simulink model "TPGCI_control_Simulation"  (R2024a)
settings: Solver=ode4  StartTime=0.0  StopTime=5  FixedStep=1e-6  RelTol=1e-3
undefined symbols (not defined in the file): DiscIntNeverNeededParam
libraries: slpidlib x3, spsThreePhaseSeriesRLCBranchLib x2, spsThreePhaseVIMeasurementLib x2, spsabctodq0Lib x2, spsDCVoltageSourceLib x1, spsGroundLib x1, spsPWMGenerator2LevelLib x1, spsThreePhaseParallelRLCBranchLib x1, spsThreePhaseSourceLib x1, spsUniversalBridgeLib x1, spsVoltageMeasurementLib x1, spsdq0toabcLib x1
settings Model: Creator=mahes  LastModifiedBy=mahes

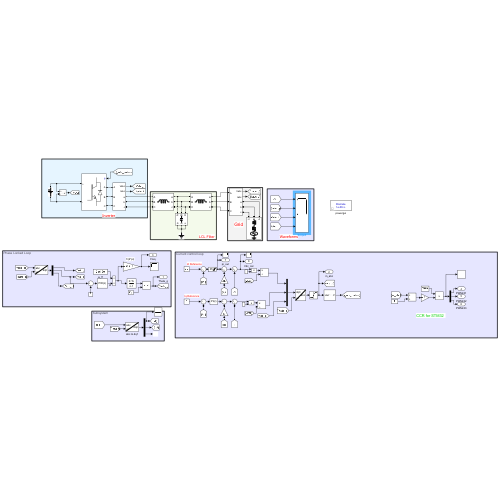
[thumbnail: Simulink's stored preview of the top-level diagram]
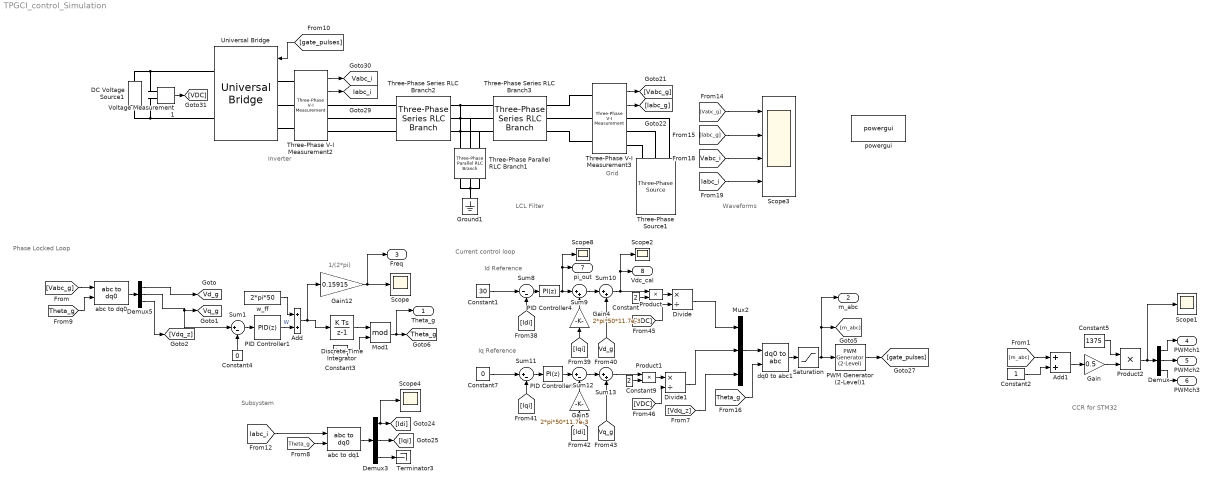
== system TPGCI_control_Simulation ==
  note: Subsystem
  note: Current control loop
  note: 1/(2*pi)
  note: Phase Locked Loop
  note: Grid
  note: Inverter
  note: Waveforms
  note: LCL Filter
  note: Id Reference
  note: Iq Reference
  note: CCR for STM32
  Add : Sum
  Add1 : Sum
  Constant : Constant  Value=2
  Constant1 : Constant  Value=30
  Constant2 : Constant
  Constant3 : Constant  Value=2*pi
  Constant4 : Constant  Value=0
  Constant5 : Constant  Value=1375
  Constant7 : Constant  Value=0
  Constant9 : Constant  Value=2
  DC Voltage Source1 : spsDCVoltageSourceLib/DC Voltage Source  Amplitude=800  Measurements=None
  Demux : Demux  Outputs=3
  Demux3 : Demux  Outputs=3
  Demux5 : Demux  Outputs=3
  Discrete-Time Integrator : DiscreteIntegrator  SampleTime=2e-5  ICPrevOutput=DiscIntNeverNeededParam  ICPrevScaledInput=DiscIntNeverNeededParam
  Divide : Product  Inputs=*/
  Divide1 : Product  Inputs=*/
  Gain : Gain  Gain=0.5
  Gain12 : Gain  Gain=0.15915
  Gain4 : Gain  Gain=2*pi*50*11.7e-3
  Gain5 : Gain  Gain=2*pi*50*11.7e-3
  Ground1 : spsGroundLib/Ground  LConnTagsString=a
  Mod1 : Math  Operator=mod
  Mux2 : Mux  Inputs=3
  PID Controller1 : slpidlib/PID Controller  Controller=PID  Form=Parallel  TimeDomain=Discrete-time  UseExternalTs=off  SampleTime=2e-5  IntegratorMethod=Forward Euler  FilterMethod=Forward Euler  ControllerParametersSource=internal  P=10  I=10000  UseKiTs=off  D=0  UseExternalDerivativeSource=off  N=100  UseFilter=on  TunerSelectOption=Transfer Function Based (PID Tuner App)  InitialConditionSource=internal  InitialConditionForIntegrator=0  InitialConditionForFilter=0  DifferentiatorICPrevScaledInput=0  ExternalReset=none  TrackingMode=off  Kt=1  LimitOutput=off  SatLimitsSource=internal  UpperSaturationLimit=inf  LowerSaturationLimit=-inf  LinearizeAsGain=on  AntiWindupMode=none  Kb=1  LimitIntegrator=off  UpperIntegratorSaturationLimit=inf  LowerIntegratorSaturationLimit=-inf  POutMin=[]  POutMax=[]  IOutMin=[]  IOutMax=[]  DOutMin=[]  DOutMax=[]  NOutMin=[]  NOutMax=[]  SumOutMin=[]  SumOutMax=[]  SaturationOutMin=[]  SaturationOutMax=[]  PParamMin=[]  PParamMax=[]  IParamMin=[]  IParamMax=[]  DParamMin=[]  DParamMax=[]  NParamMin=[]  NParamMax=[]  KbParamMin=[]  KbParamMax=[]  KtParamMin=[]  KtParamMax=[]  KbOutMin=[]  KbOutMax=[]  KtOutMin=[]  KtOutMax=[]  IntegratorOutMin=[]  IntegratorOutMax=[]  FilterOutMin=[]  FilterOutMax=[]  SumI1OutMin=[]  SumI1OutMax=[]  SumI2OutMin=[]  SumI2OutMax=[]  SumI3OutMin=[]  SumI3OutMax=[]  SumI4OutMin=[]  SumI4OutMax=[]  SumDOutMin=[]  SumDOutMax=[]  DifferentiatorOutMin=[]  DifferentiatorOutMax=[]  FilterDiffOutCoefMin=[]  FilterDiffOutCoefMax=[]  ReciprocalOutMin=[]  ReciprocalOutMax=[]  SumDenOutMin=[]  SumDenOutMax=[]  SumNumOutMin=[]  SumNumOutMax=[]  DivideOutMin=[]  DivideOutMax=[]  UdiffTsProdOutMin=[]  UdiffTsProdOutMax=[]  NTsProdOutMin=[]  NTsProdOutMax=[]  UintegralTsProdOutMin=[]  UintegralTsProdOutMax=[]  UngainTsProdOutMin=[]  UngainTsProdOutMax=[]  ClampingZeroOutDataTypeStr=Inherit: Inherit via back propagation  ClampingZeroOutMin=[]  ClampingZeroOutMax=[]  FilterDenConstantOutDataTypeStr=Inherit: Inherit via back propagation  FilterDenConstantOutMin=[]  FilterDenConstantOutMax=[]  PCopyOutDataTypeStr=Inherit: Inherit via back propagation  PCopyOutMin=[]  PCopyOutMax=[]  NCopyOutDataTypeStr=Inherit: Inherit via back propagation  NCopyOutMin=[]  NCopyOutMax=[]  IntegratorContinuousStateAttributes=''  IntegratorStateMustResolveToSignalObject=off  IntegratorRTWStateStorageClass=Auto  FilterContinuousStateAttributes=''  FilterStateMustResolveToSignalObject=off  FilterRTWStateStorageClass=Auto  ParallelPVariant=InternalParameters  IdealPVariant=Disabled  IVariant=InternalParameters  DVariant=InternalParameters  IntegratorVariant=Discrete  SatVariant=Disabled  AWVariant=Passthrough  PCopyVariant=Disabled  TRVariant=Disabled  FdbkBlocksVariant=Forward  IdealPFdbkVariant=Disabled  SatFdbkVariant=Disabled  DerivativeFilterVariant=ForwardEulerFilter  NVariant=InternalParameters  NCopyVariant=Disabled  FilterICVariant=InternalICsFilter  IntegratorICVariant=InternalICs  ExternalResetVariant=Disabled  TRSumVariant=Passthrough  SumFdbkVariant=Disabled  SumVariant=Sum_PID  TsampFilterVariant=InternalTs  TsampNgainVariant=Passthrough  TsampIntegralVariant=Disabled_SignalSpec  ExternalSaturationOutDataTypeStr=Inherit: Same as second input  DerivativeSourceVariant=ErrorSignal
  PID Controller4 : slpidlib/PID Controller  Controller=PI  Form=Parallel  TimeDomain=Discrete-time  UseExternalTs=off  SampleTime=2e-5  IntegratorMethod=Forward Euler  FilterMethod=Forward Euler  ControllerParametersSource=internal  P=1  I=100  UseKiTs=off  D=0  UseExternalDerivativeSource=off  N=100  UseFilter=on  TunerSelectOption=Transfer Function Based (PID Tuner App)  InitialConditionSource=internal  InitialConditionForIntegrator=0  InitialConditionForFilter=0  DifferentiatorICPrevScaledInput=0  ExternalReset=none  TrackingMode=off  Kt=1  LimitOutput=on  SatLimitsSource=internal  UpperSaturationLimit=10  LowerSaturationLimit=-10  LinearizeAsGain=on  AntiWindupMode=none  Kb=1  LimitIntegrator=on  UpperIntegratorSaturationLimit=10  LowerIntegratorSaturationLimit=-10  POutMin=[]  POutMax=[]  IOutMin=[]  IOutMax=[]  DOutMin=[]  DOutMax=[]  NOutMin=[]  NOutMax=[]  SumOutMin=[]  SumOutMax=[]  SaturationOutMin=[]  SaturationOutMax=[]  PParamMin=[]  PParamMax=[]  IParamMin=[]  IParamMax=[]  DParamMin=[]  DParamMax=[]  NParamMin=[]  NParamMax=[]  KbParamMin=[]  KbParamMax=[]  KtParamMin=[]  KtParamMax=[]  KbOutMin=[]  KbOutMax=[]  KtOutMin=[]  KtOutMax=[]  IntegratorOutMin=[]  IntegratorOutMax=[]  FilterOutMin=[]  FilterOutMax=[]  SumI1OutMin=[]  SumI1OutMax=[]  SumI2OutMin=[]  SumI2OutMax=[]  SumI3OutMin=[]  SumI3OutMax=[]  SumI4OutMin=[]  SumI4OutMax=[]  SumDOutMin=[]  SumDOutMax=[]  DifferentiatorOutMin=[]  DifferentiatorOutMax=[]  FilterDiffOutCoefMin=[]  FilterDiffOutCoefMax=[]  ReciprocalOutMin=[]  ReciprocalOutMax=[]  SumDenOutMin=[]  SumDenOutMax=[]  SumNumOutMin=[]  SumNumOutMax=[]  DivideOutMin=[]  DivideOutMax=[]  UdiffTsProdOutMin=[]  UdiffTsProdOutMax=[]  NTsProdOutMin=[]  NTsProdOutMax=[]  UintegralTsProdOutMin=[]  UintegralTsProdOutMax=[]  UngainTsProdOutMin=[]  UngainTsProdOutMax=[]  ClampingZeroOutDataTypeStr=Inherit: Inherit via back propagation  ClampingZeroOutMin=[]  ClampingZeroOutMax=[]  FilterDenConstantOutDataTypeStr=Inherit: Inherit via back propagation  FilterDenConstantOutMin=[]  FilterDenConstantOutMax=[]  PCopyOutDataTypeStr=Inherit: Inherit via back propagation  PCopyOutMin=[]  PCopyOutMax=[]  NCopyOutDataTypeStr=Inherit: Inherit via back propagation  NCopyOutMin=[]  NCopyOutMax=[]  IntegratorContinuousStateAttributes=''  IntegratorStateMustResolveToSignalObject=off  IntegratorRTWStateStorageClass=Auto  FilterContinuousStateAttributes=''  FilterStateMustResolveToSignalObject=off  FilterRTWStateStorageClass=Auto  ParallelPVariant=InternalParameters  IdealPVariant=Disabled  IVariant=InternalParameters  DVariant=Disabled  IntegratorVariant=Discrete  SatVariant=Enabled  AWVariant=Passthrough  PCopyVariant=Disabled  TRVariant=Disabled  FdbkBlocksVariant=Forward  IdealPFdbkVariant=Disabled  SatFdbkVariant=Disabled  DerivativeFilterVariant=Disabled  NVariant=Disabled  NCopyVariant=Disabled_SignalSpec  FilterICVariant=Disabled  IntegratorICVariant=InternalICs  ExternalResetVariant=Disabled  TRSumVariant=Passthrough  SumFdbkVariant=Disabled  SumVariant=Sum_PI  TsampFilterVariant=InternalTs  TsampNgainVariant=Passthrough  TsampIntegralVariant=Disabled_SignalSpec  ExternalSaturationOutDataTypeStr=Inherit: Same as second input  DerivativeSourceVariant=Disabled
  PID Controller5 : slpidlib/PID Controller  Controller=PI  Form=Parallel  TimeDomain=Discrete-time  UseExternalTs=off  SampleTime=2e-5  IntegratorMethod=Forward Euler  FilterMethod=Forward Euler  ControllerParametersSource=internal  P=1  I=100  UseKiTs=off  D=0  UseExternalDerivativeSource=off  N=100  UseFilter=on  TunerSelectOption=Transfer Function Based (PID Tuner App)  InitialConditionSource=internal  InitialConditionForIntegrator=0  InitialConditionForFilter=0  DifferentiatorICPrevScaledInput=0  ExternalReset=none  TrackingMode=off  Kt=1  LimitOutput=off  SatLimitsSource=internal  UpperSaturationLimit=inf  LowerSaturationLimit=-inf  LinearizeAsGain=on  AntiWindupMode=none  Kb=1  LimitIntegrator=off  UpperIntegratorSaturationLimit=inf  LowerIntegratorSaturationLimit=-inf  POutMin=[]  POutMax=[]  IOutMin=[]  IOutMax=[]  DOutMin=[]  DOutMax=[]  NOutMin=[]  NOutMax=[]  SumOutMin=[]  SumOutMax=[]  SaturationOutMin=[]  SaturationOutMax=[]  PParamMin=[]  PParamMax=[]  IParamMin=[]  IParamMax=[]  DParamMin=[]  DParamMax=[]  NParamMin=[]  NParamMax=[]  KbParamMin=[]  KbParamMax=[]  KtParamMin=[]  KtParamMax=[]  KbOutMin=[]  KbOutMax=[]  KtOutMin=[]  KtOutMax=[]  IntegratorOutMin=[]  IntegratorOutMax=[]  FilterOutMin=[]  FilterOutMax=[]  SumI1OutMin=[]  SumI1OutMax=[]  SumI2OutMin=[]  SumI2OutMax=[]  SumI3OutMin=[]  SumI3OutMax=[]  SumI4OutMin=[]  SumI4OutMax=[]  SumDOutMin=[]  SumDOutMax=[]  DifferentiatorOutMin=[]  DifferentiatorOutMax=[]  FilterDiffOutCoefMin=[]  FilterDiffOutCoefMax=[]  ReciprocalOutMin=[]  ReciprocalOutMax=[]  SumDenOutMin=[]  SumDenOutMax=[]  SumNumOutMin=[]  SumNumOutMax=[]  DivideOutMin=[]  DivideOutMax=[]  UdiffTsProdOutMin=[]  UdiffTsProdOutMax=[]  NTsProdOutMin=[]  NTsProdOutMax=[]  UintegralTsProdOutMin=[]  UintegralTsProdOutMax=[]  UngainTsProdOutMin=[]  UngainTsProdOutMax=[]  ClampingZeroOutDataTypeStr=Inherit: Inherit via back propagation  ClampingZeroOutMin=[]  ClampingZeroOutMax=[]  FilterDenConstantOutDataTypeStr=Inherit: Inherit via back propagation  FilterDenConstantOutMin=[]  FilterDenConstantOutMax=[]  PCopyOutDataTypeStr=Inherit: Inherit via back propagation  PCopyOutMin=[]  PCopyOutMax=[]  NCopyOutDataTypeStr=Inherit: Inherit via back propagation  NCopyOutMin=[]  NCopyOutMax=[]  IntegratorContinuousStateAttributes=''  IntegratorStateMustResolveToSignalObject=off  IntegratorRTWStateStorageClass=Auto  FilterContinuousStateAttributes=''  FilterStateMustResolveToSignalObject=off  FilterRTWStateStorageClass=Auto  ParallelPVariant=InternalParameters  IdealPVariant=Disabled  IVariant=InternalParameters  DVariant=Disabled  IntegratorVariant=Discrete  SatVariant=Disabled  AWVariant=Passthrough  PCopyVariant=Disabled  TRVariant=Disabled  FdbkBlocksVariant=Forward  IdealPFdbkVariant=Disabled  SatFdbkVariant=Disabled  DerivativeFilterVariant=Disabled  NVariant=Disabled  NCopyVariant=Disabled_SignalSpec  FilterICVariant=Disabled  IntegratorICVariant=InternalICs  ExternalResetVariant=Disabled  TRSumVariant=Passthrough  SumFdbkVariant=Disabled  SumVariant=Sum_PI  TsampFilterVariant=InternalTs  TsampNgainVariant=Passthrough  TsampIntegralVariant=Disabled_SignalSpec  ExternalSaturationOutDataTypeStr=Inherit: Same as second input  DerivativeSourceVariant=Disabled
  PWM Generator (2-Level)1 : spsPWMGenerator2LevelLib/PWM Generator (2-Level)  ModulatorType=Three-phase bridge (6 pulses)  ModulatorMode=Unsynchronized  Fc=10e3  Pc=90  nF=27  MinMax="[ -1  1 ]"  SamplingTechnique=Natural  ModulatingSignals=off  m=0.8  Freq=60  Phase=0  Ts=0  ShowCarrierOutport=off
  Product : Product
  Product1 : Product
  Product2 : Product
  Saturation : Saturate  UpperLimit=0.95  LowerLimit=-0.95
  Scope{,1..2,4,8} (5 alike) : Scope
  Scope3 : Scope  NumInputPorts=4
  Sum1 : Sum  Inputs=|+-
  Sum10 : Sum  Inputs=|++
  Sum11 : Sum  Inputs=|+-
  Sum12 : Sum  Inputs=|+-
  Sum13 : Sum  Inputs=|++
  Sum8 : Sum  Inputs=|--
  Sum9 : Sum  Inputs=|++
  Terminator3 : Terminator
  Three-Phase Parallel RLC Branch1 : spsThreePhaseParallelRLCBranchLib/Three-Phase Parallel RLC Branch  LConnTagsString=A|B|C  RConnTagsString=A|B|C  BranchType=C  Resistance=1  Inductance=1e-3  Capacitance=5.986e-6  Measurements=None
  Three-Phase Series RLC Branch2 : spsThreePhaseSeriesRLCBranchLib/Three-Phase Series RLC Branch  LConnTagsString=A|B|C  RConnTagsString=A|B|C  BranchType=L  Resistance=1  Inductance=9e-3  Capacitance=1e-6  Measurements=None
  Three-Phase Series RLC Branch3 : spsThreePhaseSeriesRLCBranchLib/Three-Phase Series RLC Branch  LConnTagsString=A|B|C  RConnTagsString=A|B|C  BranchType=L  Resistance=1  Inductance=2.7e-3  Capacitance=1e-6  Measurements=None
  Three-Phase V-I Measurement2 : spsThreePhaseVIMeasurementLib/Three-Phase V-I Measurement  VoltageMeasurement=phase-to-ground  SetLabelV=off  LabelV=Vabc  Vpu=off  VpuLL=off  CurrentMeasurement=yes  SetLabelI=off  LabelI=Iabc  Ipu=off  Pbase=100e6  Vbase=500e3  OutputType=Complex  PhasorSimulation=off  PSBequivalent=0
  Three-Phase V-I Measurement3 : spsThreePhaseVIMeasurementLib/Three-Phase V-I Measurement  VoltageMeasurement=phase-to-ground  SetLabelV=off  LabelV=Vabc  Vpu=off  VpuLL=off  CurrentMeasurement=yes  SetLabelI=off  LabelI=Iabc  Ipu=off  Pbase=100e6  Vbase=500e3  OutputType=Complex  PhasorSimulation=off  PSBequivalent=0
  Three-Phase Source1 : spsThreePhaseSourceLib/Three-Phase Source  InternalConnection=Yg  VoltagePhases=off  Voltage=400  PhaseAngle=0  Voltage_phases=[25e3 25e3 25e3]/sqrt(3)  PhaseAngles_phases=[0 -120 +120]  Frequency=50  NonIdealSource=on  SpecifyImpedance=off  Resistance=0.0001e-3  Inductance=0.0001e-9  ShortCircuitLevel=100e6  BaseVoltage=400  XRratio=7  BusType=swing  Pref=10e3  Qref=0  Prefabc=[10e3, 10e3, 10e3]  Qrefabc=[0, 0, 0]  Qmin=-inf  Qmax=inf
  Universal Bridge : spsUniversalBridgeLib/Universal Bridge  Arms=3  SnubberResistance=1e5  SnubberCapacitance=inf  Device=IGBT / Diodes  Ron=1e-3  Lon=0  ForwardVoltages="[  0  0  ]"  ForwardVoltage=0  GTOparameters=[ 10e-6 , 20e-6 ]  IGBTparameters=[ 1e-6 , 2e-6 ]  Measurements=None  Measurements_2=None  converterType=Rectifier
  Voltage Measurement1 : spsVoltageMeasurementLib/Voltage Measurement  PhasorSimulation=off  OutputType=Complex  PSBequivalent=0
  abc to dq0 : spsabctodq0Lib/abc to dq0  Alignment=90 degrees behind phase A axis
  abc to dq1 : spsabctodq0Lib/abc to dq0  Alignment=90 degrees behind phase A axis
  dq0 to abc1 : spsdq0toabcLib/dq0 to abc  Alignment=90 degrees behind phase A axis
  powergui : sps_lib/powergui  Priority=1  SimulationMode=Discrete  SampleTime=1e-6  frequency=60  Iterations=50  frequencyindice=0  Pbase=100e6  ErrMax=1e-4  UnitsV=kV  UnitsW=MW  buscounter=0  FunctionMessages=off  echomessages=off  EnableUseOfTLC=off  CurrentSourceSwitches=off  DisableSnubberDevices=off  DisableRonSwitches=off  DisableVfSwitches=off  DisplayEquations=off  AutomaticDiscreteSolvers=off  SolverType=Tustin/Backward Euler (TBE)  Interpol=off  ExternalGateDelay=off  methode=off  Ts=100  x0status=blocks  SPID=on  SwTol=0  HookPort=off  NonlinearTolerance=1e-4  nMaxIteration=100  ContinueOnMaxIteration=off  RestoreLinks=warning  ResistiveCurrentMeasurement=off  Frange=[0:2:500]  Ylog=off  Xlog=on  ShowGrid=off  save=off  variable=ZData  structure=0  ZoomFFT=off  StartTime=0.0  cycles=1  DisplayStyle=1  fundamental=60  FreqAxis=off  MaxFrequency=1000  frequencyindicesteady=1  RmsSteady=1  display=off
  w_ff : Constant  Value=2*pi*50
  Theta_g : Outport
  m_abc : Outport  Port=2
  Freq : Outport  Port=3
  PWMch1 : Outport  Port=4
  PWMch2 : Outport  Port=5
  PWMch3 : Outport  Port=6
  pi_out : Outport  Port=7
  Vdc_cal : Outport  Port=8
  tag scope: Iabc_i=global, Theta_g=global, Vabc_i=global, Vd_g=global, Vq_g=global
  wires:
  Demux5/3 -> [Vdq_z]
  Discrete-Time Integrator/1 -> Mod1/1
  Constant3/1 -> Mod1/2
  Demux5/2 -> Sum1/1, [Vq_g]
  Constant4/1 -> Sum1/2
  Mod1/1 -> [Theta_g], Theta_g/1
  Sum1/1 -> PID Controller1/1
  Demux5/1 -> [Vd_g]
  PID Controller1/1 -> Add/2  "W"
  w_ff/1 -> Add/1
  Add/1 -> Gain12/1, Discrete-Time Integrator/1
  Gain12/1 -> Freq/1, Scope/1
  [Iabc_g] -> Scope3/2
  Three-Phase V-I Measurement2/1 -> [Vabc_i]
  [Iabc_i] -> Scope3/4
  Three-Phase V-I Measurement3/1 -> [Vabc_g]
  [Vabc_g] -> Scope3/1
  [Vabc_i] -> Scope3/3
  Three-Phase V-I Measurement2/2 -> [Iabc_i]
  Three-Phase V-I Measurement3/2 -> [Iabc_g]
  [gate_pulses] -> Universal Bridge/1
  abc to dq0/1 -> Demux5/1
  [Theta_g] -> abc to dq0/2
  Voltage Measurement1/1 -> [VDC]
  [Vabc_g] -> abc to dq0/1
  [Iqi] -> Sum11/2
  [Idi] -> Gain5/1
  Product1/1 -> Divide1/1
  [VDC] -> Divide1/2
  Gain4/1 -> Sum9/2
  Constant1/1 -> Sum8/1
  Sum13/1 -> Product1/1
  Mux2/1 -> dq0 to abc1/1
  [Idi] -> Sum8/2
  PID Controller5/1 -> Sum12/1
  Sum9/1 -> Sum10/1
  Constant/1 -> Product/2
  Sum8/1 -> PID Controller4/1
  Gain5/1 -> Sum12/2
  [Vdq_z] -> Mux2/3
  Sum11/1 -> PID Controller5/1
  PID Controller4/1 -> Sum9/1, pi_out/1, Scope8/1
  Divide/1 -> Mux2/1
  [VDC] -> Divide/2
  Constant9/1 -> Product1/2
  Divide1/1 -> Mux2/2
  [Vd_g] -> Sum10/2
  [Theta_g] -> dq0 to abc1/2
  Saturation/1 -> m_abc/1, [m_abc], PWM Generator (2-Level)1/1
  PWM Generator (2-Level)1/1 -> [gate_pulses]
  Constant7/1 -> Sum11/1
  dq0 to abc1/1 -> Saturation/1
  [Vq_g] -> Sum13/2
  Sum12/1 -> Sum13/1
  Sum10/1 -> Product/1, Scope2/1, Vdc_cal/1
  Product/1 -> Divide/1
  [Iqi] -> Gain4/1
  [m_abc] -> Add1/1
  Constant2/1 -> Add1/2
  Constant5/1 -> Product2/1
  Product2/1 -> Scope1/1, Demux/1
  Demux/1 -> PWMch1/1
  Demux/2 -> PWMch2/1
  Demux/3 -> PWMch3/1
  Add1/1 -> Gain/1
  Gain/1 -> Product2/2
  [Iabc_i] -> abc to dq1/1
  Demux3/3 -> Terminator3/1
  abc to dq1/1 -> Demux3/1
  Demux3/2 -> [Iqi]
  Demux3/1 -> Scope4/1, [Idi]
  [Theta_g] -> abc to dq1/2
  connections:
  Three-Phase Series RLC Branch2/RConn3 -- Three-Phase Series RLC Branch3/LConn3 -- Three-Phase Parallel RLC Branch1/LConn3
  Three-Phase Parallel RLC Branch1/RConn2 -- Three-Phase Parallel RLC Branch1/RConn1 -- Three-Phase Parallel RLC Branch1/RConn3 -- Ground1/LConn1
  Three-Phase Series RLC Branch2/RConn2 -- Three-Phase Series RLC Branch3/LConn2 -- Three-Phase Parallel RLC Branch1/LConn2
  Three-Phase Series RLC Branch2/RConn1 -- Three-Phase Series RLC Branch3/LConn1 -- Three-Phase Parallel RLC Branch1/LConn1
  Universal Bridge/LConn2 -- Three-Phase V-I Measurement2/LConn2
  DC Voltage Source1/LConn1 -- Universal Bridge/RConn2 -- Voltage Measurement1/LConn2
  Three-Phase V-I Measurement2/RConn2 -- Three-Phase Series RLC Branch2/LConn2
  Universal Bridge/LConn1 -- Three-Phase V-I Measurement2/LConn1
  Three-Phase V-I Measurement3/RConn1 -- Three-Phase Source1/RConn1
  Three-Phase Series RLC Branch3/RConn3 -- Three-Phase V-I Measurement3/LConn3
  Three-Phase V-I Measurement2/RConn1 -- Three-Phase Series RLC Branch2/LConn1
  Universal Bridge/LConn3 -- Three-Phase V-I Measurement2/LConn3
  Three-Phase Series RLC Branch3/RConn1 -- Three-Phase V-I Measurement3/LConn1
  Three-Phase V-I Measurement2/RConn3 -- Three-Phase Series RLC Branch2/LConn3
  Three-Phase Series RLC Branch3/RConn2 -- Three-Phase V-I Measurement3/LConn2
  Three-Phase V-I Measurement3/RConn3 -- Three-Phase Source1/RConn3
  DC Voltage Source1/RConn1 -- Voltage Measurement1/LConn1 -- Universal Bridge/RConn1
  Three-Phase V-I Measurement3/RConn2 -- Three-Phase Source1/RConn2
